simulink model "DDDRmode"  (R2020a)
settings: Solver=VariableStepAuto  StartTime=0.0  StopTime=10.0  RelTol=1e-3
settings Model: Creator=Liam  LastModifiedBy=Liam

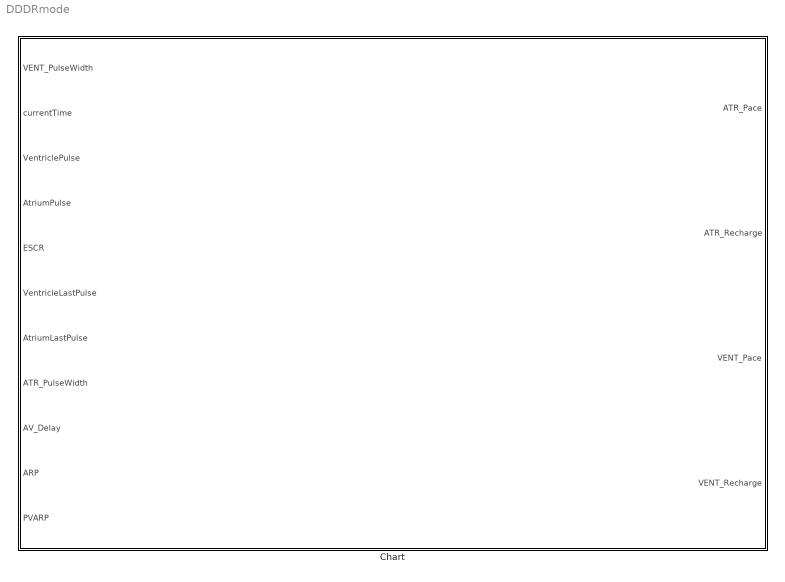
== system DDDRmode ==
  Chart : Stateflow chart  TreatAsAtomicUnit=on

== stateflow chart DDDRmode/Chart ==
  note: Need to implenment a no skip pace if it is in the deadzone (use ARP)
  state ATR_Recharge
    entry:
    ATR_Recharge=2;
  state ATR_Recharge_init
    entry:
    ATR_Pace=false;
    VENT_Pace=false;
    ATR_Recharge=1;
    VENT_Recharge=0;
  state ATR_Pace
    entry:
    ATR_Pace=true;
    ATR_Recharge=0;
  state VENT_Recharge_init
    entry:
    ATR_Pace=false;
    VENT_Pace=false;
    VENT_Recharge=1;
    ATR_Recharge=0;
  state VENT_Pace
    entry:
    VENT_Pace=true;
    VENT_Recharge=0;
  state VENT_Recharge
    entry:
    VENT_Recharge=2;
  note: there is the possiblility that the stateflow gets stuck at the VENT_Recharge and ATR_Recharge states if the heart is pacing normally
  state ATR_Recharge_init1 [commented out]
    entry:
    ATR_Pace=false;
    VENT_Pace=false;
    ATR_Recharge=1;
  state ATR_Recharge1 [commented out]
    entry:
    ATR_Recharge=2;
    note: another possiblility
  state VENT_Recharge_init1 [commented out]
    entry:
    ATR_Pace=false;
    VENT_Pace=false;
    VENT_Recharge=1;
  state VENT_Recharge1 [commented out]
    entry:
    VENT_Recharge=2;
  state VENT_Pace1 [commented out]
    entry:
    VENT_Pace=true;
    VENT_Recharge=0;
  state ATR_Pace1 [commented out]
    entry:
    ATR_Pace=true;
    ATR_Recharge=0;
  (default) -> ATR_Recharge_init
  ATR_Recharge_init -> ATR_Recharge
  ATR_Recharge -> ATR_Pace [order 1] : [currentTime-AtriumLastPulse>ESCR]
  ATR_Pace -> VENT_Recharge_init : [after(ATR_PulseWidth,msec)]
  VENT_Pace -> ATR_Recharge_init : [after(VENT_PulseWidth,msec)]
  VENT_Recharge -> ATR_Recharge_init [order 2] : [VentriclePulse==true && currentTime-(AtriumLastPulse+AV_Delay)>PVARP]
  ATR_Recharge -> VENT_Recharge_init [order 2] : [AtriumPulse==true && currentTime-AtriumLastPulse>ARP]
  VENT_Recharge_init -> VENT_Recharge
  VENT_Recharge -> VENT_Pace [order 1] : [currentTime-(AtriumLastPulse+AV_Delay)>ESCR]
  (default) -> ATR_Recharge_init1 [commented out]
  (default) -> VENT_Recharge_init1 [commented out]
  ATR_Recharge_init1 -> ATR_Recharge1 [commented out]
  ATR_Pace1 -> ATR_Recharge_init1 [commented out] : [after(ATR_PulseWidth,msec)]
  VENT_Recharge_init1 -> VENT_Recharge1 [commented out]
  ATR_Recharge1 -> ATR_Pace1 [commented out] : [currentTime-AtriumLastPulse>ESCR]
  VENT_Recharge1 -> VENT_Pace1 [commented out] : [currentTime-VentricleLastPulse>ESCR]
  VENT_Pace1 -> VENT_Recharge_init1 [commented out] : [after(VENT_PulseWidth, msec)]
  data: VENT_PulseWidth input; currentTime input; ATR_Pace output; ATR_Recharge output; VENT_Pace output; VENT_Recharge output; VentriclePulse input; AtriumPulse input; ESCR input; VentricleLastPulse input; AtriumLastPulse input; ATR_PulseWidth input; AV_Delay input; ARP input; PVARP input
